simulink model "Ass3"  (R2018b)
settings: Solver=VariableStepAuto  StartTime=0.0  StopTime=10.0  RelTol=1e-3
undefined symbols (not defined in the file or in its folder): sys_p
libraries: cstblocks x1
settings Model: Creator=bigfoot  LastModifiedBy=bigfoot

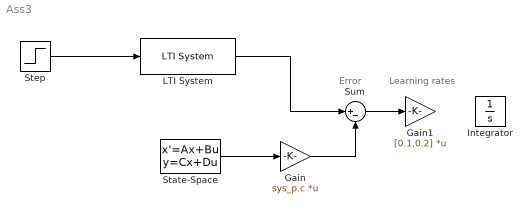
== system Ass3 ==
  note: Learning rates
  note: Error
  Gain : Gain  Gain=sys_p.c  Multiplication=Matrix(K*u)
  Gain1 : Gain  Gain=[0.1,0.2]  Multiplication=Matrix(K*u)
  Integrator : Integrator
  LTI System : cstblocks/LTI System  sys=Model  IC=[]
  State-Space : StateSpace  A=sys_p.a  B=sys_p.b  C=eye(2)  D=[0;0]  InitialCondition=0
  Step : Step  SampleTime=0
  Sum : Sum  Inputs=|+-
  wires:
  Step/1 -> LTI System/1
  State-Space/1 -> Gain/1
  Gain/1 -> Sum/2
  LTI System/1 -> Sum/1
  Sum/1 -> Gain1/1
